simulink model "feature_model"  (R2023b)
settings: Solver=FixedStepDiscrete  StartTime=0.0  StopTime=inf  FixedStep=0.1  RelTol=1e-3
settings Model: Creator=RDONASC1  LastModifiedBy=RDONASC1
settings OptimizationCC: DefaultParameterBehavior=Inlined  EnhancedBackFolding=on  PassReuseOutputArgsAs=Individual arguments  ZeroExternalMemoryAtStartup=off  ZeroInternalMemoryAtStartup=off  OptimizeBlockOrder=speed  DifferentSizesBufferReuse=on  OptimizationCustomize=off  EfficientTunableParamExpr=on
settings DebuggingCC: ParameterTunabilityLossMsg=error
settings SFSimCC: MATLABDynamicMemAlloc=off
settings RTWCC: Description=Embedded Coder  SystemTargetFile=ert.tlc  TemplateMakefile=ert_default_tmf
settings CodeAppCC: ForceParamTrailComments=on  IgnoreCustomStorageClasses=off  OperatorAnnotations=on  SimulinkDataObjDesc=on  SFDataObjDesc=on  InsertBlockDesc=on
settings ERTTargetCC: TargetLangStandard=C99 (ISO)  GenerateSampleERTMain=on  InlinedParameterPlacement=NonHierarchical  ERTCustomFileTemplate=example_file_process.tlc

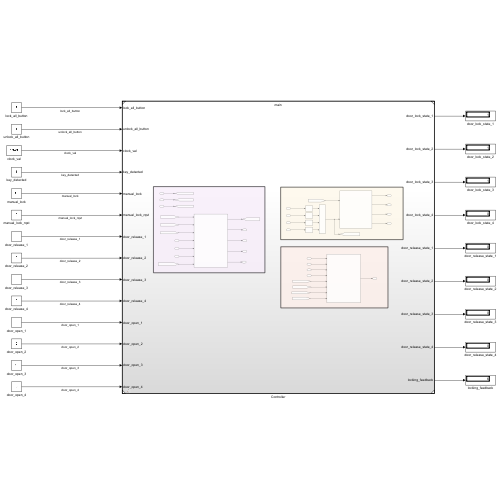
[thumbnail: Simulink's stored preview of the top-level diagram]
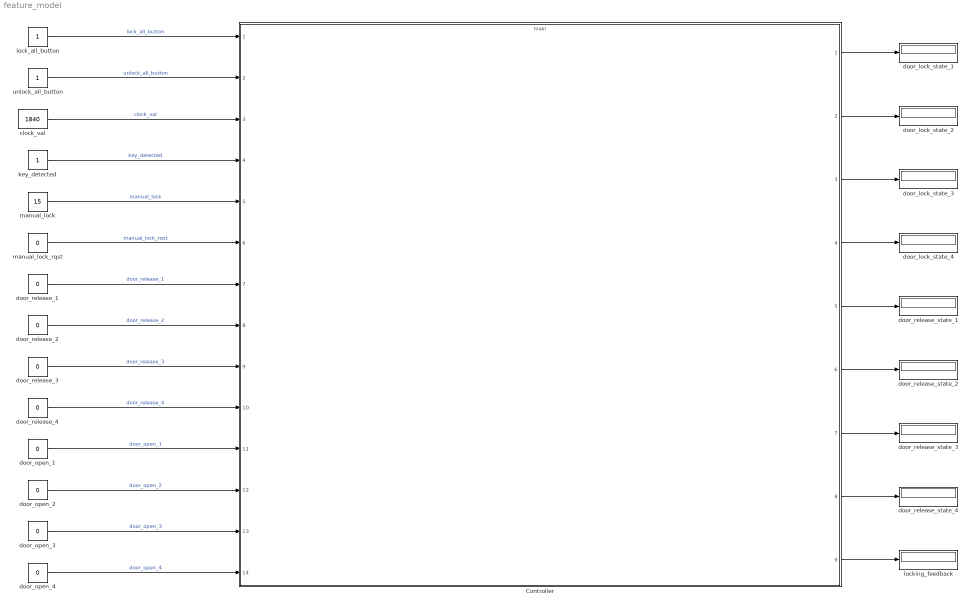
== system feature_model ==
  Controller : ModelReference  ModelNameDialog=main.slx  SimulationMode=Normal  ModelReferenceVersion=1.121
  clock_val : Constant  Value=1840  OutDataTypeStr=uint64
  door_lock_state_{1..4} (4 alike) : Display
  door_open_{1..4} (4 alike) : Constant  Value=0  OutDataTypeStr=uint8
  door_release_{1..4} (4 alike) : Constant  Value=0  OutMin=0  OutMax=1  OutDataTypeStr=uint8
  door_release_state_{1..4} (4 alike) : Display
  key_detected : Constant  OutDataTypeStr=uint8
  lock_all_button : Constant  OutDataTypeStr=uint8
  locking_feedback : Display
  manual_lock : Constant  Value=15  OutDataTypeStr=uint8
  manual_lock_rqst : Constant  Value=0  OutDataTypeStr=uint8
  unlock_all_button : Constant  OutDataTypeStr=uint8
  wires:
  lock_all_button/1 -> Controller/1  "lock_all_button"
  unlock_all_button/1 -> Controller/2  "unlock_all_button"
  key_detected/1 -> Controller/4  "key_detected"
  Controller/1 -> door_lock_state_1/1
  clock_val/1 -> Controller/3  "clock_val"
  manual_lock/1 -> Controller/5  "manual_lock"
  Controller/9 -> locking_feedback/1
  Controller/5 -> door_release_state_1/1
  Controller/4 -> door_lock_state_4/1
  Controller/3 -> door_lock_state_3/1
  Controller/2 -> door_lock_state_2/1
  Controller/8 -> door_release_state_4/1
  Controller/7 -> door_release_state_3/1
  Controller/6 -> door_release_state_2/1
  manual_lock_rqst/1 -> Controller/6  "manual_lock_rqst"
  door_release_1/1 -> Controller/7  "door_release_1"
  door_release_2/1 -> Controller/8  "door_release_2"
  door_release_3/1 -> Controller/9  "door_release_3"
  door_release_4/1 -> Controller/10  "door_release_4"
  door_open_1/1 -> Controller/11  "door_open_1"
  door_open_2/1 -> Controller/12  "door_open_2"
  door_open_3/1 -> Controller/13  "door_open_3"
  door_open_4/1 -> Controller/14  "door_open_4"
